simulink model "model"  (R2014a)
settings: Solver=ode45  StartTime=0.0  StopTime=100.0  MaxStep=2  RelTol=1e-3
undefined symbols (not defined in the file): t0, u0, ug
libraries: simulink x1
settings Model: Creator=dariush  LastModifiedBy=dariush

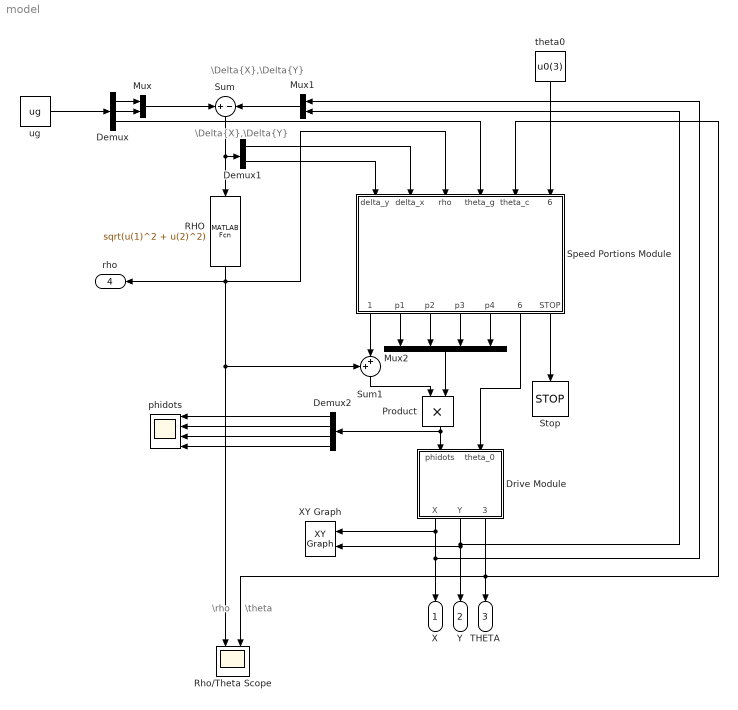
== system model ==
  note: \theta
  note: \rho
  note: \Delta{X},\Delta{Y}
  note: \Delta{X},\Delta{Y}
  Demux : Demux  Outputs=3
  Demux1 : Demux  Outputs=2
  Demux2 : Demux
  Drive Module : Subsystem
  Mux : Mux  Inputs=2
  Mux1 : Mux  Inputs=2
  Mux2 : Mux
  Product : Product
  RHO : MATLABFcn  MATLABFcn=sqrt(u(1)^2 + u(2)^2)
  Rho/Theta Scope : Scope  NumInputPorts=2
      settings: YMin=-5~-5  YMax=5~5
  Speed Portions Module : MATLAB Function  TreatAsAtomicUnit=on
  Stop : Stop
  Sum : Sum  Inputs=+|-
  Sum1 : Sum  Inputs=++|
  XY Graph : simulink/Sinks/XY Graph  xmin=-10  xmax=10  ymin=-10  ymax=10  st=-1
  phidots : Scope  NumInputPorts=4
      settings: TimeRange=80  YMin=-5~-5~-5~-5  YMax=5~5~5~5
  theta0 : Constant  Value=u0(3)
  ug : Constant  Value=ug
  X : Outport
  Y : Outport  Port=2
  THETA : Outport  Port=3
  rho : Outport  Port=4
  wires:
  Drive Module/1(X) -> XY Graph/1, Mux1/1, X/1
  ug/1 -> Demux/1
  Demux/1 -> Mux/1
  Demux/2 -> Mux/2
  Mux/1 -> Sum/1
  Mux1/1 -> Sum/2
  Sum/1 -> RHO/1, Demux1/1
  Mux2/1 -> Product/2
  Demux1/1 -> Speed Portions Module/2(delta_x)
  Demux1/2 -> Speed Portions Module/1(delta_y)
  Speed Portions Module/5(p4) -> Mux2/4
  Speed Portions Module/4(p3) -> Mux2/3
  Speed Portions Module/3(p2) -> Mux2/2
  Speed Portions Module/2(p1) -> Mux2/1
  Demux/3 -> Speed Portions Module/4(theta_g)
  Speed Portions Module/7(STOP) -> Stop/1
  Drive Module/2(Y) -> XY Graph/2, Y/1, Mux1/2
  Sum1/1 -> Product/1
  Speed Portions Module/1(rho_epsilon) -> Sum1/2
  Speed Portions Module/6(theta_0out) -> Drive Module/2(theta_0)
  RHO/1 -> Rho/Theta Scope/1, Sum1/1, Speed Portions Module/3(rho), rho/1
  Drive Module/3(THETA) -> Rho/Theta Scope/2, Speed Portions Module/5(theta_c), THETA/1
  theta0/1 -> Speed Portions Module/6(theta_0in)
  Product/1 -> Drive Module/1(phidots), Demux2/1
  Demux2/1 -> phidots/1
  Demux2/2 -> phidots/2
  Demux2/3 -> phidots/3
  Demux2/4 -> phidots/4

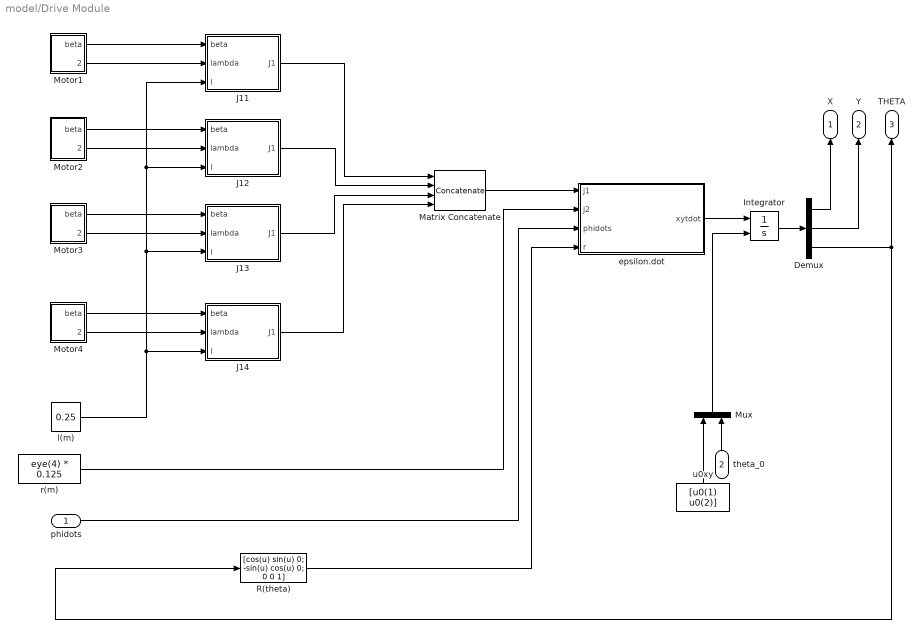
== system model/Drive Module ==
  phidots : Inport
  theta_0 : Inport  Port=2
  Demux : Demux  Outputs=3
  Integrator : Integrator  InitialConditionSource=external  InitialCondition=[u0(1) u0(2) t0]
  J11 : Subsystem
  J12 : Subsystem
  J13 : Subsystem
  J14 : Subsystem
  Matrix Concatenate : Concatenate  NumInputs=4  Mode=Multidimensional array
  Motor1 : Subsystem
  Motor2 : Subsystem
  Motor3 : Subsystem
  Motor4 : Subsystem
  Mux : Mux  Inputs=2
  R(theta) : MATLABFcn  MATLABFcn=[cos(u) sin(u) 0; -sin(u) cos(u) 0; 0 0 1]  Output1D=off
  epsilon.dot : MATLAB Function  TreatAsAtomicUnit=on
  l(m) : Constant  Value=0.25
  r(m) : Constant  Value=eye(4) * 0.125
  u0xy : Constant  Value=[u0(1) u0(2)]
  X : Outport
  Y : Outport  Port=2
  THETA : Outport  Port=3
  wires:
  Motor1/1(beta) -> J11/1(beta)
  Motor1/2(lambda) -> J11/2(lambda)
  Motor2/1(beta) -> J12/1(beta)
  Motor2/2(lambda) -> J12/2(lambda)
  Motor3/1(beta) -> J13/1(beta)
  Motor3/2(lambda) -> J13/2(lambda)
  Motor4/1(beta) -> J14/1(beta)
  Motor4/2(lambda) -> J14/2(lambda)
  l(m)/1 -> J11/3("l "), J12/3(l), J13/3(l), J14/3(l)
  r(m)/1 -> epsilon.dot/2(j2)
  Demux/2 -> Y/1
  J11/1(J1) -> Matrix Concatenate/1
  Demux/1 -> X/1
  J12/1(J1) -> Matrix Concatenate/2
  J13/1(J1) -> Matrix Concatenate/3
  J14/1(J1) -> Matrix Concatenate/4
  epsilon.dot/1(xytdot) -> Integrator/1
  Integrator/1 -> Demux/1
  Matrix Concatenate/1 -> epsilon.dot/1(j1)
  R(theta)/1 -> epsilon.dot/4(r)
  Demux/3 -> THETA/1, R(theta)/1
  phidots/1 -> epsilon.dot/3(phidots)
  Mux/1 -> Integrator/2
  u0xy/1 -> Mux/1
  theta_0/1 -> Mux/2

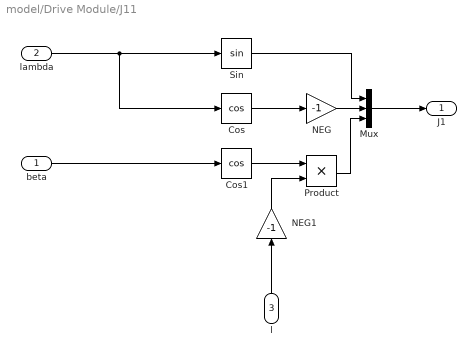
== system model/Drive Module/J11 ==
  beta : Inport
  lambda : Inport  Port=2
  "l " : Inport  Port=3
  Cos : Trigonometry  Operator=cos
  Cos1 : Trigonometry  Operator=cos
  Mux : Mux  Inputs=3
  NEG : Gain  Gain=-1
  NEG1 : Gain  Gain=-1
  Product : Product
  "Sin " : Trigonometry
  J1 : Outport  PortDimensions=[1,3]
  wires:
  Cos1/1 -> Product/1
  NEG/1 -> Mux/2
  Mux/1 -> J1/1
  Cos/1 -> NEG/1
  "Sin "/1 -> Mux/1
  beta/1 -> Cos1/1
  lambda/1 -> Cos/1, "Sin "/1
  "l "/1 -> NEG1/1
  NEG1/1 -> Product/2
  Product/1 -> Mux/3

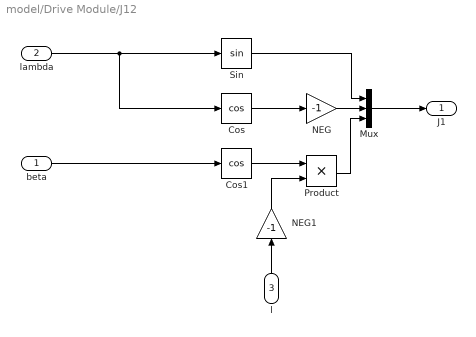
== system model/Drive Module/J12 ==
  beta : Inport
  lambda : Inport  Port=2
  l : Inport  Port=3
  Cos : Trigonometry  Operator=cos
  Cos1 : Trigonometry  Operator=cos
  Mux : Mux  Inputs=3
  NEG : Gain  Gain=-1
  NEG1 : Gain  Gain=-1
  Product : Product
  "Sin " : Trigonometry
  J1 : Outport  PortDimensions=[1,3]
  wires:
  Cos1/1 -> Product/1
  NEG/1 -> Mux/2
  Mux/1 -> J1/1
  Cos/1 -> NEG/1
  "Sin "/1 -> Mux/1
  beta/1 -> Cos1/1
  lambda/1 -> Cos/1, "Sin "/1
  l/1 -> NEG1/1
  Product/1 -> Mux/3
  NEG1/1 -> Product/2

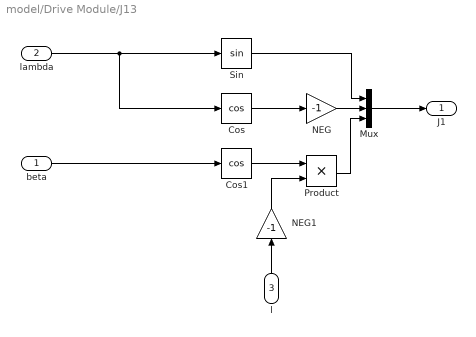
== system model/Drive Module/J13 ==
  beta : Inport
  lambda : Inport  Port=2
  l : Inport  Port=3
  Cos : Trigonometry  Operator=cos
  Cos1 : Trigonometry  Operator=cos
  Mux : Mux  Inputs=3
  NEG : Gain  Gain=-1
  NEG1 : Gain  Gain=-1
  Product : Product
  "Sin " : Trigonometry
  J1 : Outport  PortDimensions=[1,3]
  wires:
  Cos1/1 -> Product/1
  NEG/1 -> Mux/2
  Mux/1 -> J1/1
  Cos/1 -> NEG/1
  "Sin "/1 -> Mux/1
  beta/1 -> Cos1/1
  lambda/1 -> Cos/1, "Sin "/1
  l/1 -> NEG1/1
  Product/1 -> Mux/3
  NEG1/1 -> Product/2

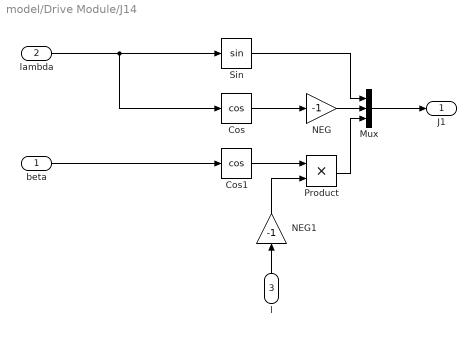
== system model/Drive Module/J14 ==
  beta : Inport
  lambda : Inport  Port=2
  l : Inport  Port=3
  Cos : Trigonometry  Operator=cos
  Cos1 : Trigonometry  Operator=cos
  Mux : Mux  Inputs=3
  NEG : Gain  Gain=-1
  NEG1 : Gain  Gain=-1
  Product : Product
  "Sin " : Trigonometry
  J1 : Outport  PortDimensions=[1,3]
  wires:
  Cos1/1 -> Product/1
  NEG/1 -> Mux/2
  Mux/1 -> J1/1
  Cos/1 -> NEG/1
  "Sin "/1 -> Mux/1
  beta/1 -> Cos1/1
  lambda/1 -> Cos/1, "Sin "/1
  l/1 -> NEG1/1
  Product/1 -> Mux/3
  NEG1/1 -> Product/2

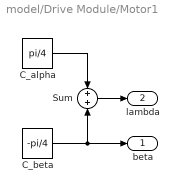
== system model/Drive Module/Motor1 ==
  C_alpha : Constant  Value=pi/4
  C_beta : Constant  Value=-pi/4
  Sum : Sum  Inputs=+|+
  beta : Outport
  lambda : Outport  Port=2
  wires:
  C_beta/1 -> beta/1, Sum/2
  C_alpha/1 -> Sum/1
  Sum/1 -> lambda/1

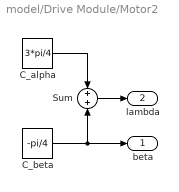
== system model/Drive Module/Motor2 ==
  C_alpha : Constant  Value=3*pi/4
  C_beta : Constant  Value=-pi/4
  Sum : Sum  Inputs=+|+
  beta : Outport
  lambda : Outport  Port=2
  wires:
  C_beta/1 -> beta/1, Sum/2
  C_alpha/1 -> Sum/1
  Sum/1 -> lambda/1

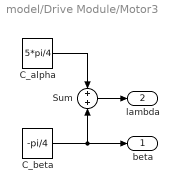
== system model/Drive Module/Motor3 ==
  C_alpha : Constant  Value=5*pi/4
  C_beta : Constant  Value=-pi/4
  Sum : Sum  Inputs=+|+
  beta : Outport
  lambda : Outport  Port=2
  wires:
  C_beta/1 -> beta/1, Sum/2
  C_alpha/1 -> Sum/1
  Sum/1 -> lambda/1

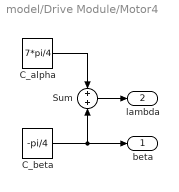
== system model/Drive Module/Motor4 ==
  C_alpha : Constant  Value=7*pi/4
  C_beta : Constant  Value=-pi/4
  Sum : Sum  Inputs=+|+
  beta : Outport
  lambda : Outport  Port=2
  wires:
  C_beta/1 -> beta/1, Sum/2
  C_alpha/1 -> Sum/1
  Sum/1 -> lambda/1

== matlab function model/Drive Module/epsilon.dot ==
  data: j1 input; j2 input; phidots input; xytdot output; r input
function xytdot = epsilon_dot(j1, j2, phidots, r)
% coder.extrinsic('assignin');
% assignin('base', 'r',  r);
% assignin('base', 'j1', j1);
% assignin('base', 'pr',  pinv(r));
% assignin('base', 'pj1', pinv(j1));
% assignin('base', 'j2', j2);
% assignin('base', 'phidots', phidots);
xytdot = pinv(r) * pinv(j1) * j2 * phidots;

== matlab function model/Speed Portions Module ==
  data: delta_y input; delta_x input; rho input; theta_g input; theta_c input; rho_epsilon output; p1 output; p2 output; p3 output; p4 output; theta_0out output; STOP output; theta_0in input
function [rho_epsilon, p1, p2, p3, p4, theta_0out, STOP] = SPM(delta_y, delta_x, rho, theta_g, theta_c, theta_0in)
    % init all output to zero
    [p1, p2, p3, p4, STOP, rho_epsilon, theta_0out] = deal(0);
    theta_c = theta_c + theta_0in;
    is_near_point = (rho <= 0.05);
    if(is_near_point && abs(angdiff(theta_g, theta_c)) <= pi/180)
        STOP = 1;
        return;
    end
    if (~is_near_point)
        [p1, p2, p3, p4] = correct_point(delta_y, delta_x);
    else
        [p1, p2, p3, p4] = correct_theta(theta_g , theta_c);
        if(rho == 0)
            rho_epsilon = 1;
        end
    end
end
function [p1, p2, p3, p4] = correct_point(delta_y, delta_x)
    at = atan2(delta_y, delta_x);
    cxy = round2(sin(at), 1e-1);
    cyx = round2(cos(at), 1e-1);
    p1 = -cxy;
    p2 = cyx;
    p3 = cxy;
    p4 = -cyx;
    disp('> Location Correction');
end
function [p1, p2, p3, p4] = correct_theta(theta_g , theta_c)
    [p1, p2, p3, p4] = deal(0);
    diff = angdiff(theta_g , theta_c);
    if(abs(diff) > pi/180)
        [p1, p2, p3, p4] = deal(-diff * 4);
        disp('> Angel Correction');
    end
end
